simulink model "ThdRwRtStCalib"  (R2024b)
settings: Solver=FixedStepDiscrete  StartTime=0.0  StopTime=10.0  FixedStep=0.01  RelTol=1e-3
model workspace (MAT data in the model file):
  KeSMSwAcsMd7ThdRwRtStBkReclnUpwdDnwdPosMax_Val : Simulink.Parameter (value not decoded)
  KeSMSwAcsMd7ThdRwRtStBkReclnUpwdDnwdPosMin_Val : Simulink.Parameter (value not decoded)
  KeSMSwAcsMd7ThdRwRtStBkReclnUpwdDnwdPos_Val : Simulink.Parameter (value not decoded)
  KeSMSwAcsMd7ThdRwRtStCshnFldUpwdDnwdPosMax_Val : Simulink.Parameter (value not decoded)
  KeSMSwAcsMd7ThdRwRtStCshnFldUpwdDnwdPosMin_Val : Simulink.Parameter (value not decoded)
  KeSMSwAcsMd7ThdRwRtStCshnFldUpwdDnwdPos_Val : Simulink.Parameter (value not decoded)
  KeSMSwAcsMd7ThdRwRtStFrwdBkwdPosMax_Val : Simulink.Parameter (value not decoded)
  KeSMSwAcsMd7ThdRwRtStFrwdBkwdPosMin_Val : Simulink.Parameter (value not decoded)
  KeSMSwAcsMd7ThdRwRtStFrwdBkwdPos_Val : Simulink.Parameter (value not decoded)
symbols that are objects in the model workspace (value not decoded): KeSMSwAcsMd7ThdRwRtStBkReclnUpwdDnwdPos_Val, KeSMSwAcsMd7ThdRwRtStBkReclnUpwdDnwdPosMax_Val, KeSMSwAcsMd7ThdRwRtStBkReclnUpwdDnwdPosMin_Val, KeSMSwAcsMd7ThdRwRtStCshnFldUpwdDnwdPos_Val, KeSMSwAcsMd7ThdRwRtStCshnFldUpwdDnwdPosMax_Val, KeSMSwAcsMd7ThdRwRtStCshnFldUpwdDnwdPosMin_Val, KeSMSwAcsMd7ThdRwRtStFrwdBkwdPos_Val, KeSMSwAcsMd7ThdRwRtStFrwdBkwdPosMax_Val, KeSMSwAcsMd7ThdRwRtStFrwdBkwdPosMin_Val
undefined symbols (not defined in the file or in its folder): KeSMSw6sAcsEntryThdRwRtStBkReclnUpwdDnwdPos_Val, KeSMSw6sAcsEntryThdRwRtStBkReclnUpwdDnwdPosMax_Val, KeSMSw6sAcsEntryThdRwRtStBkReclnUpwdDnwdPosMin_Val, KeSMSw6sAcsEntryThdRwRtStCshnFldUpwdDnwdPos_Val, KeSMSw6sAcsEntryThdRwRtStCshnFldUpwdDnwdPosMax_Val, KeSMSw6sAcsEntryThdRwRtStCshnFldUpwdDnwdPosMin_Val, KeSMSw6sAcsEntryThdRwRtStFrwdBkwdPos_Val, KeSMSw6sAcsEntryThdRwRtStFrwdBkwdPosMax_Val, KeSMSw6sAcsEntryThdRwRtStFrwdBkwdPosMin_Val, KeSMSw6SAcsMd56ThdRwRtStBkReclnUpwdDnwdPos_Val, KeSMSw6SAcsMd56ThdRwRtStBkReclnUpwdDnwdPosMax_Val, KeSMSw6SAcsMd56ThdRwRtStBkReclnUpwdDnwdPosMin_Val, KeSMSw6SAcsMd56ThdRwRtStFrwdBkwdPos_Val, KeSMSw6SAcsMd56ThdRwRtStFrwdBkwdPosMax_Val, KeSMSw6SAcsMd56ThdRwRtStFrwdBkwdPosMin_Val, KeSMSw6SAcsMd57ThdRwRtStBkReclnUpwdDnwdPos_Val, KeSMSw6SAcsMd57ThdRwRtStBkReclnUpwdDnwdPosMax_Val, KeSMSw6SAcsMd57ThdRwRtStBkReclnUpwdDnwdPosMin_Val, KeSMSw6SAcsMd57ThdRwRtStFrwdBkwdPos_Val, KeSMSw6SAcsMd57ThdRwRtStFrwdBkwdPosMax_Val, KeSMSw6SAcsMd57ThdRwRtStFrwdBkwdPosMin_Val, KeSMSw6sFamilyMdThdRwRtStFrwdBkwdPos_Val, KeSMSw6sFamilyMdThdRwRtStFrwdBkwdPosMax_Val, KeSMSw6sFamilyMdThdRwRtStFrwdBkwdPosMin_Val, KeSMSw6sFamilyRMdThdRwRtStFrwdBkwdPos_Val, KeSMSw6sFamilyRMdThdRwRtStFrwdBkwdPosMax_Val, KeSMSw6sFamilyRMdThdRwRtStFrwdBkwdPosMin_Val, KeSMSw6sLugThdRwRtStBkReclnUpwdDnwdPos_Val, KeSMSw6sLugThdRwRtStBkReclnUpwdDnwdPosMax_Val, KeSMSw6sLugThdRwRtStBkReclnUpwdDnwdPosMin_Val, KeSMSw6sLugThdRwRtStCshnFldUpwdDnwdPos_Val, KeSMSw6sLugThdRwRtStCshnFldUpwdDnwdPosMax_Val, KeSMSw6sLugThdRwRtStCshnFldUpwdDnwdPosMin_Val, KeSMSw6sLugThdRwRtStFrwdBkwdPos_Val, KeSMSw6sLugThdRwRtStFrwdBkwdPosMax_Val, KeSMSw6sLugThdRwRtStFrwdBkwdPosMin_Val, KeSMSw6sVIPThdRwRtStBkReclnUpwdDnwdPos_Val, KeSMSw6sVIPThdRwRtStBkReclnUpwdDnwdPosMax_Val, KeSMSw6sVIPThdRwRtStBkReclnUpwdDnwdPosMin_Val, KeSMSw6sVIPThdRwRtStFrwdBkwdPos_Val, KeSMSw6sVIPThdRwRtStFrwdBkwdPosMax_Val, KeSMSw6sVIPThdRwRtStFrwdBkwdPosMin_Val, KeSMSwAcsEntryThdRwRtStBkReclnUpwdDnwdPos_Val, KeSMSwAcsEntryThdRwRtStBkReclnUpwdDnwdPosMax_Val, KeSMSwAcsEntryThdRwRtStBkReclnUpwdDnwdPosMin_Val, KeSMSwAcsEntryThdRwRtStCshnFldUpwdDnwdPos_Val, KeSMSwAcsEntryThdRwRtStCshnFldUpwdDnwdPosMax_Val, KeSMSwAcsEntryThdRwRtStCshnFldUpwdDnwdPosMin_Val, KeSMSwAcsEntryThdRwRtStFrwdBkwdPos_Val, KeSMSwAcsEntryThdRwRtStFrwdBkwdPosMax_Val, KeSMSwAcsEntryThdRwRtStFrwdBkwdPosMin_Val, KeSMSwAcsMd53ThdRwRtBkReclnUpwdDnwdPos_Val, KeSMSwAcsMd53ThdRwRtBkReclnUpwdDnwdPosMax_Val, KeSMSwAcsMd53ThdRwRtBkReclnUpwdDnwdPosMin_Val, KeSMSwAcsMd53ThdRwRtFldUpwdDnwdPos_Val, KeSMSwAcsMd53ThdRwRtFldUpwdDnwdPosMax_Val, KeSMSwAcsMd53ThdRwRtFldUpwdDnwdPosMin_Val, KeSMSwAcsMd56ThdRwRtStBkReclnUpwdDnwdPos_Val, KeSMSwAcsMd56ThdRwRtStBkReclnUpwdDnwdPosMax_Val, KeSMSwAcsMd56ThdRwRtStBkReclnUpwdDnwdPosMin_Val ... (+33)
libraries: TrgtPosSelcLib x18
(part 2 of 3)

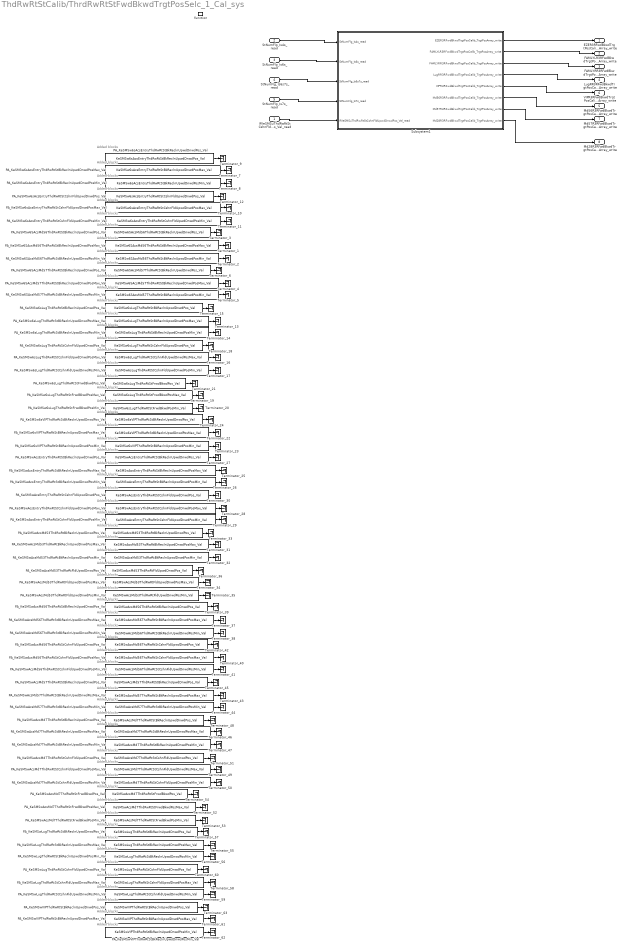
== system ThdRwRtStCalib/ThrdRwRtStFwdBkwdTrgtPosSelc_1_Cal_sys ==
  note: Added blocks
  note: Added blocks
  note: Added blocks
  note: Added blocks
  note: Added blocks
  note: Added blocks
  note: Added blocks
  note: Added blocks
  note: Added blocks
  note: Added blocks
  note: Added blocks
  note: Added blocks
  note: Added blocks
  note: Added blocks
  note: Added blocks
  note: Added blocks
  note: Added blocks
  note: Added blocks
  note: Added blocks
  note: Added blocks
  note: Added blocks
  note: Added blocks
  note: Added blocks
  note: Added blocks
  note: Added blocks
  note: Added blocks
  note: Added blocks
  note: Added blocks
  note: Added blocks
  note: Added blocks
  note: Added blocks
  note: Added blocks
  note: Added blocks
  note: Added blocks
  note: Added blocks
  note: Added blocks
  note: Added blocks
  note: Added blocks
  note: Added blocks
  note: Added blocks
  note: Added blocks
  note: Added blocks
  note: Added blocks
  note: Added blocks
  note: Added blocks
  note: Added blocks
  note: Added blocks
  note: Added blocks
  note: Added blocks
  note: Added blocks
  note: Added blocks
  note: Added blocks
  note: Added blocks
  note: Added blocks
  note: Added blocks
  note: Added blocks
  note: Added blocks
  note: Added blocks
  note: Added blocks
  note: Added blocks
  note: Added blocks
  note: Added blocks
  note: Added blocks
  IfVeSMSuThdRwRtStCshnFldUpwdDnwdPos_Val_read : Inport
  StNumFlg_Is4s_read : Inport  Port=2
  StNumFlg_Is6s_read : Inport  Port=3
  StNumFlg_Is6s7s_read : Inport  Port=4
  StNumFlg_Is7s_read : Inport  Port=5
  function : TriggerPort  TriggerType=function-call  IsSimulinkFunction=on  FunctionName=ThrdRwRtStFwdBkwdTrgtPosSelc_1_Cal  VariantControl=(inherit)
  PA_KeSMSw6SAcsMd56ThdRwRtStBkReclnUpwdDnwdPosMax_Val : Constant  Value=KeSMSw6SAcsMd56ThdRwRtStBkReclnUpwdDnwdPosMax_Val
  PA_KeSMSw6SAcsMd56ThdRwRtStBkReclnUpwdDnwdPosMin_Val : Constant  Value=KeSMSw6SAcsMd56ThdRwRtStBkReclnUpwdDnwdPosMin_Val
  PA_KeSMSw6SAcsMd56ThdRwRtStBkReclnUpwdDnwdPos_Val : Constant  Value=KeSMSw6SAcsMd56ThdRwRtStBkReclnUpwdDnwdPos_Val
  PA_KeSMSw6SAcsMd57ThdRwRtStBkReclnUpwdDnwdPosMax_Val : Constant  Value=KeSMSw6SAcsMd57ThdRwRtStBkReclnUpwdDnwdPosMax_Val
  PA_KeSMSw6SAcsMd57ThdRwRtStBkReclnUpwdDnwdPosMin_Val : Constant  Value=KeSMSw6SAcsMd57ThdRwRtStBkReclnUpwdDnwdPosMin_Val
  PA_KeSMSw6SAcsMd57ThdRwRtStBkReclnUpwdDnwdPos_Val : Constant  Value=KeSMSw6SAcsMd57ThdRwRtStBkReclnUpwdDnwdPos_Val
  PA_KeSMSw6sAcsEntryThdRwRtStBkReclnUpwdDnwdPosMax_Val : Constant  Value=KeSMSw6sAcsEntryThdRwRtStBkReclnUpwdDnwdPosMax_Val
  PA_KeSMSw6sAcsEntryThdRwRtStBkReclnUpwdDnwdPosMin_Val : Constant  Value=KeSMSw6sAcsEntryThdRwRtStBkReclnUpwdDnwdPosMin_Val
  PA_KeSMSw6sAcsEntryThdRwRtStBkReclnUpwdDnwdPos_Val : Constant  Value=KeSMSw6sAcsEntryThdRwRtStBkReclnUpwdDnwdPos_Val
  PA_KeSMSw6sAcsEntryThdRwRtStCshnFldUpwdDnwdPosMax_Val : Constant  Value=KeSMSw6sAcsEntryThdRwRtStCshnFldUpwdDnwdPosMax_Val
  PA_KeSMSw6sAcsEntryThdRwRtStCshnFldUpwdDnwdPosMin_Val : Constant  Value=KeSMSw6sAcsEntryThdRwRtStCshnFldUpwdDnwdPosMin_Val
  PA_KeSMSw6sAcsEntryThdRwRtStCshnFldUpwdDnwdPos_Val : Constant  Value=KeSMSw6sAcsEntryThdRwRtStCshnFldUpwdDnwdPos_Val
  PA_KeSMSw6sLugThdRwRtStBkReclnUpwdDnwdPosMax_Val : Constant  Value=KeSMSw6sLugThdRwRtStBkReclnUpwdDnwdPosMax_Val
  PA_KeSMSw6sLugThdRwRtStBkReclnUpwdDnwdPosMin_Val : Constant  Value=KeSMSw6sLugThdRwRtStBkReclnUpwdDnwdPosMin_Val
  PA_KeSMSw6sLugThdRwRtStBkReclnUpwdDnwdPos_Val : Constant  Value=KeSMSw6sLugThdRwRtStBkReclnUpwdDnwdPos_Val
  PA_KeSMSw6sLugThdRwRtStCshnFldUpwdDnwdPosMax_Val : Constant  Value=KeSMSw6sLugThdRwRtStCshnFldUpwdDnwdPosMax_Val
  PA_KeSMSw6sLugThdRwRtStCshnFldUpwdDnwdPosMin_Val : Constant  Value=KeSMSw6sLugThdRwRtStCshnFldUpwdDnwdPosMin_Val
  PA_KeSMSw6sLugThdRwRtStCshnFldUpwdDnwdPos_Val : Constant  Value=KeSMSw6sLugThdRwRtStCshnFldUpwdDnwdPos_Val
  PA_KeSMSw6sLugThdRwRtStFrwdBkwdPosMax_Val : Constant  Value=KeSMSw6sLugThdRwRtStFrwdBkwdPosMax_Val
  PA_KeSMSw6sLugThdRwRtStFrwdBkwdPosMin_Val : Constant  Value=KeSMSw6sLugThdRwRtStFrwdBkwdPosMin_Val
  PA_KeSMSw6sLugThdRwRtStFrwdBkwdPos_Val : Constant  Value=KeSMSw6sLugThdRwRtStFrwdBkwdPos_Val
  PA_KeSMSw6sVIPThdRwRtStBkReclnUpwdDnwdPosMax_Val : Constant  Value=KeSMSw6sVIPThdRwRtStBkReclnUpwdDnwdPosMax_Val
  PA_KeSMSw6sVIPThdRwRtStBkReclnUpwdDnwdPosMin_Val : Constant  Value=KeSMSw6sVIPThdRwRtStBkReclnUpwdDnwdPosMin_Val
  PA_KeSMSw6sVIPThdRwRtStBkReclnUpwdDnwdPos_Val : Constant  Value=KeSMSw6sVIPThdRwRtStBkReclnUpwdDnwdPos_Val
  PA_KeSMSwAcsEntryThdRwRtStBkReclnUpwdDnwdPosMax_Val : Constant  Value=KeSMSwAcsEntryThdRwRtStBkReclnUpwdDnwdPosMax_Val
  PA_KeSMSwAcsEntryThdRwRtStBkReclnUpwdDnwdPosMin_Val : Constant  Value=KeSMSwAcsEntryThdRwRtStBkReclnUpwdDnwdPosMin_Val
  PA_KeSMSwAcsEntryThdRwRtStBkReclnUpwdDnwdPos_Val : Constant  Value=KeSMSwAcsEntryThdRwRtStBkReclnUpwdDnwdPos_Val
  PA_KeSMSwAcsEntryThdRwRtStCshnFldUpwdDnwdPosMax_Val : Constant  Value=KeSMSwAcsEntryThdRwRtStCshnFldUpwdDnwdPosMax_Val
  PA_KeSMSwAcsEntryThdRwRtStCshnFldUpwdDnwdPosMin_Val : Constant  Value=KeSMSwAcsEntryThdRwRtStCshnFldUpwdDnwdPosMin_Val
  PA_KeSMSwAcsEntryThdRwRtStCshnFldUpwdDnwdPos_Val : Constant  Value=KeSMSwAcsEntryThdRwRtStCshnFldUpwdDnwdPos_Val
  PA_KeSMSwAcsMd53ThdRwRtBkReclnUpwdDnwdPosMax_Val : Constant  Value=KeSMSwAcsMd53ThdRwRtBkReclnUpwdDnwdPosMax_Val
  PA_KeSMSwAcsMd53ThdRwRtBkReclnUpwdDnwdPosMin_Val : Constant  Value=KeSMSwAcsMd53ThdRwRtBkReclnUpwdDnwdPosMin_Val
  PA_KeSMSwAcsMd53ThdRwRtBkReclnUpwdDnwdPos_Val : Constant  Value=KeSMSwAcsMd53ThdRwRtBkReclnUpwdDnwdPos_Val
  PA_KeSMSwAcsMd53ThdRwRtFldUpwdDnwdPosMax_Val : Constant  Value=KeSMSwAcsMd53ThdRwRtFldUpwdDnwdPosMax_Val
  PA_KeSMSwAcsMd53ThdRwRtFldUpwdDnwdPosMin_Val : Constant  Value=KeSMSwAcsMd53ThdRwRtFldUpwdDnwdPosMin_Val
  PA_KeSMSwAcsMd53ThdRwRtFldUpwdDnwdPos_Val : Constant  Value=KeSMSwAcsMd53ThdRwRtFldUpwdDnwdPos_Val
  PA_KeSMSwAcsMd56ThdRwRtStBkReclnUpwdDnwdPosMax_Val : Constant  Value=KeSMSwAcsMd56ThdRwRtStBkReclnUpwdDnwdPosMax_Val
  PA_KeSMSwAcsMd56ThdRwRtStBkReclnUpwdDnwdPosMin_Val : Constant  Value=KeSMSwAcsMd56ThdRwRtStBkReclnUpwdDnwdPosMin_Val
  PA_KeSMSwAcsMd56ThdRwRtStBkReclnUpwdDnwdPos_Val : Constant  Value=KeSMSwAcsMd56ThdRwRtStBkReclnUpwdDnwdPos_Val
  PA_KeSMSwAcsMd56ThdRwRtStCshnFldUpwdDnwdPosMax_Val : Constant  Value=KeSMSwAcsMd56ThdRwRtStCshnFldUpwdDnwdPosMax_Val
  PA_KeSMSwAcsMd56ThdRwRtStCshnFldUpwdDnwdPosMin_Val : Constant  Value=KeSMSwAcsMd56ThdRwRtStCshnFldUpwdDnwdPosMin_Val
  PA_KeSMSwAcsMd56ThdRwRtStCshnFldUpwdDnwdPos_Val : Constant  Value=KeSMSwAcsMd56ThdRwRtStCshnFldUpwdDnwdPos_Val
  PA_KeSMSwAcsMd57ThdRwRtStBkReclnUpwdDnwdPosMax_Val : Constant  Value=KeSMSwAcsMd57ThdRwRtStBkReclnUpwdDnwdPosMax_Val
  PA_KeSMSwAcsMd57ThdRwRtStBkReclnUpwdDnwdPosMin_Val : Constant  Value=KeSMSwAcsMd57ThdRwRtStBkReclnUpwdDnwdPosMin_Val
  PA_KeSMSwAcsMd57ThdRwRtStBkReclnUpwdDnwdPos_Val : Constant  Value=KeSMSwAcsMd57ThdRwRtStBkReclnUpwdDnwdPos_Val
  PA_KeSMSwAcsMd7ThdRwRtStBkReclnUpwdDnwdPosMax_Val : Constant  Value=KeSMSwAcsMd7ThdRwRtStBkReclnUpwdDnwdPosMax_Val
  PA_KeSMSwAcsMd7ThdRwRtStBkReclnUpwdDnwdPosMin_Val : Constant  Value=KeSMSwAcsMd7ThdRwRtStBkReclnUpwdDnwdPosMin_Val
  PA_KeSMSwAcsMd7ThdRwRtStBkReclnUpwdDnwdPos_Val : Constant  Value=KeSMSwAcsMd7ThdRwRtStBkReclnUpwdDnwdPos_Val
  PA_KeSMSwAcsMd7ThdRwRtStCshnFldUpwdDnwdPosMax_Val : Constant  Value=KeSMSwAcsMd7ThdRwRtStCshnFldUpwdDnwdPosMax_Val
  PA_KeSMSwAcsMd7ThdRwRtStCshnFldUpwdDnwdPosMin_Val : Constant  Value=KeSMSwAcsMd7ThdRwRtStCshnFldUpwdDnwdPosMin_Val
  PA_KeSMSwAcsMd7ThdRwRtStCshnFldUpwdDnwdPos_Val : Constant  Value=KeSMSwAcsMd7ThdRwRtStCshnFldUpwdDnwdPos_Val
  PA_KeSMSwAcsMd7ThdRwRtStFrwdBkwdPosMax_Val : Constant  Value=KeSMSwAcsMd7ThdRwRtStFrwdBkwdPosMax_Val
  PA_KeSMSwAcsMd7ThdRwRtStFrwdBkwdPosMin_Val : Constant  Value=KeSMSwAcsMd7ThdRwRtStFrwdBkwdPosMin_Val
  PA_KeSMSwAcsMd7ThdRwRtStFrwdBkwdPos_Val : Constant  Value=KeSMSwAcsMd7ThdRwRtStFrwdBkwdPos_Val
  PA_KeSMSwLugThdRwRtStBkReclnUpwdDnwdPosMax_Val : Constant  Value=KeSMSwLugThdRwRtStBkReclnUpwdDnwdPosMax_Val
  PA_KeSMSwLugThdRwRtStBkReclnUpwdDnwdPosMin_Val : Constant  Value=KeSMSwLugThdRwRtStBkReclnUpwdDnwdPosMin_Val
  PA_KeSMSwLugThdRwRtStBkReclnUpwdDnwdPos_Val : Constant  Value=KeSMSwLugThdRwRtStBkReclnUpwdDnwdPos_Val
  PA_KeSMSwLugThdRwRtStCshnFldUpwdDnwdPosMax_Val : Constant  Value=KeSMSwLugThdRwRtStCshnFldUpwdDnwdPosMax_Val
  PA_KeSMSwLugThdRwRtStCshnFldUpwdDnwdPosMin_Val : Constant  Value=KeSMSwLugThdRwRtStCshnFldUpwdDnwdPosMin_Val
  PA_KeSMSwLugThdRwRtStCshnFldUpwdDnwdPos_Val : Constant  Value=KeSMSwLugThdRwRtStCshnFldUpwdDnwdPos_Val
  PA_KeSMSwVIPThdRwRtStBkReclnUpwdDnwdPosMax_Val : Constant  Value=KeSMSwVIPThdRwRtStBkReclnUpwdDnwdPosMax_Val
  PA_KeSMSwVIPThdRwRtStBkReclnUpwdDnwdPosMin_Val : Constant  Value=KeSMSwVIPThdRwRtStBkReclnUpwdDnwdPosMin_Val
  PA_KeSMSwVIPThdRwRtStBkReclnUpwdDnwdPos_Val : Constant  Value=KeSMSwVIPThdRwRtStBkReclnUpwdDnwdPos_Val
  Subsystem1 : Subsystem
  Terminator_{1..63} (63 alike) : Terminator
  EZER3RFwdBkwdTrgtPosCalib_TrgtPosArray_write : Outport  VectorParamsAs1DForOutWhenUnconnected=off
  FAMLYLR3RFwdBkwdTrgtPosCalib_TrgtPosArray_write : Outport  Port=2  VectorParamsAs1DForOutWhenUnconnected=off
  FAMLYRR3RFwdBkwdTrgtPosCalib_TrgtPosArray_write : Outport  Port=3  VectorParamsAs1DForOutWhenUnconnected=off
  LugRR3RFwdBkwdTrgtPosCalib_TrgtPosArray_write : Outport  Port=4  VectorParamsAs1DForOutWhenUnconnected=off
  Md56R3RFwdBkwdTrgtPosCalib_TrgtPosArray_write : Outport  Port=5  VectorParamsAs1DForOutWhenUnconnected=off
  VIPR3RFwdBkwdTrgtPosCalib_TrgtPosArray_write : Outport  Port=6  VectorParamsAs1DForOutWhenUnconnected=off
  Md57R3RFwdBkwdTrgtPosCalib_TrgtPosArray_write : Outport  Port=7  VectorParamsAs1DForOutWhenUnconnected=off
  Md28R3RFwdBkwdTrgtPosCalib_TrgtPosArray_write : Outport  Port=8  VectorParamsAs1DForOutWhenUnconnected=off
      settings: EnsureOutportIsVirtual=on
  wires:
  Subsystem1/1(EZER3RFwdBkwdTrgtPosCalib_TrgtPosArray_write) -> EZER3RFwdBkwdTrgtPosCalib_TrgtPosArray_write/1
  Subsystem1/2(FAMLYLR3RFwdBkwdTrgtPosCalib_TrgtPosArray_write) -> FAMLYLR3RFwdBkwdTrgtPosCalib_TrgtPosArray_write/1
  Subsystem1/3(FAMLYRR3RFwdBkwdTrgtPosCalib_TrgtPosArray_write) -> FAMLYRR3RFwdBkwdTrgtPosCalib_TrgtPosArray_write/1
  Subsystem1/4(LugRR3RFwdBkwdTrgtPosCalib_TrgtPosArray_write) -> LugRR3RFwdBkwdTrgtPosCalib_TrgtPosArray_write/1
  Subsystem1/5(VIPR3RFwdBkwdTrgtPosCalib_TrgtPosArray_write) -> VIPR3RFwdBkwdTrgtPosCalib_TrgtPosArray_write/1
  Subsystem1/6(Md56R3RFwdBkwdTrgtPosCalib_TrgtPosArray_write) -> Md56R3RFwdBkwdTrgtPosCalib_TrgtPosArray_write/1
  Subsystem1/7(Md57R3RFwdBkwdTrgtPosCalib_TrgtPosArray_write) -> Md57R3RFwdBkwdTrgtPosCalib_TrgtPosArray_write/1
  StNumFlg_Is4s_read/1 -> Subsystem1/1(StNumFlg_Is4s_read)
  StNumFlg_Is6s_read/1 -> Subsystem1/2(StNumFlg_Is6s_read)
  StNumFlg_Is6s7s_read/1 -> Subsystem1/3(StNumFlg_Is6s7s_read)
  StNumFlg_Is7s_read/1 -> Subsystem1/4(StNumFlg_Is7s_read)
  IfVeSMSuThdRwRtStCshnFldUpwdDnwdPos_Val_read/1 -> Subsystem1/5(IfVeSMSuThdRwRtStCshnFldUpwdDnwdPos_Val_read)
  Subsystem1/8(Md28R3RFwdBkwdTrgtPosCalib_TrgtPosArray_write) -> Md28R3RFwdBkwdTrgtPosCalib_TrgtPosArray_write/1
  PA_KeSMSw6SAcsMd56ThdRwRtStBkReclnUpwdDnwdPosMax_Val/1 -> Terminator_1/1
  PA_KeSMSw6SAcsMd56ThdRwRtStBkReclnUpwdDnwdPosMin_Val/1 -> Terminator_2/1
  PA_KeSMSw6SAcsMd56ThdRwRtStBkReclnUpwdDnwdPos_Val/1 -> Terminator_3/1
  PA_KeSMSw6SAcsMd57ThdRwRtStBkReclnUpwdDnwdPosMax_Val/1 -> Terminator_4/1
  PA_KeSMSw6SAcsMd57ThdRwRtStBkReclnUpwdDnwdPosMin_Val/1 -> Terminator_5/1
  PA_KeSMSw6SAcsMd57ThdRwRtStBkReclnUpwdDnwdPos_Val/1 -> Terminator_6/1
  PA_KeSMSw6sAcsEntryThdRwRtStBkReclnUpwdDnwdPosMax_Val/1 -> Terminator_7/1
  PA_KeSMSw6sAcsEntryThdRwRtStBkReclnUpwdDnwdPosMin_Val/1 -> Terminator_8/1
  PA_KeSMSw6sAcsEntryThdRwRtStBkReclnUpwdDnwdPos_Val/1 -> Terminator_9/1
  PA_KeSMSw6sAcsEntryThdRwRtStCshnFldUpwdDnwdPosMax_Val/1 -> Terminator_10/1
  PA_KeSMSw6sAcsEntryThdRwRtStCshnFldUpwdDnwdPosMin_Val/1 -> Terminator_11/1
  PA_KeSMSw6sAcsEntryThdRwRtStCshnFldUpwdDnwdPos_Val/1 -> Terminator_12/1
  PA_KeSMSw6sLugThdRwRtStBkReclnUpwdDnwdPosMax_Val/1 -> Terminator_13/1
  PA_KeSMSw6sLugThdRwRtStBkReclnUpwdDnwdPosMin_Val/1 -> Terminator_14/1
  PA_KeSMSw6sLugThdRwRtStBkReclnUpwdDnwdPos_Val/1 -> Terminator_15/1
  PA_KeSMSw6sLugThdRwRtStCshnFldUpwdDnwdPosMax_Val/1 -> Terminator_16/1
  PA_KeSMSw6sLugThdRwRtStCshnFldUpwdDnwdPosMin_Val/1 -> Terminator_17/1
  PA_KeSMSw6sLugThdRwRtStCshnFldUpwdDnwdPos_Val/1 -> Terminator_18/1
  PA_KeSMSw6sLugThdRwRtStFrwdBkwdPosMax_Val/1 -> Terminator_19/1
  PA_KeSMSw6sLugThdRwRtStFrwdBkwdPosMin_Val/1 -> Terminator_20/1
  PA_KeSMSw6sLugThdRwRtStFrwdBkwdPos_Val/1 -> Terminator_21/1
  PA_KeSMSw6sVIPThdRwRtStBkReclnUpwdDnwdPosMax_Val/1 -> Terminator_22/1
  PA_KeSMSw6sVIPThdRwRtStBkReclnUpwdDnwdPosMin_Val/1 -> Terminator_23/1
  PA_KeSMSw6sVIPThdRwRtStBkReclnUpwdDnwdPos_Val/1 -> Terminator_24/1
  PA_KeSMSwAcsEntryThdRwRtStBkReclnUpwdDnwdPosMax_Val/1 -> Terminator_25/1
  PA_KeSMSwAcsEntryThdRwRtStBkReclnUpwdDnwdPosMin_Val/1 -> Terminator_26/1
  PA_KeSMSwAcsEntryThdRwRtStBkReclnUpwdDnwdPos_Val/1 -> Terminator_27/1
  PA_KeSMSwAcsEntryThdRwRtStCshnFldUpwdDnwdPosMax_Val/1 -> Terminator_28/1
  PA_KeSMSwAcsEntryThdRwRtStCshnFldUpwdDnwdPosMin_Val/1 -> Terminator_29/1
  PA_KeSMSwAcsEntryThdRwRtStCshnFldUpwdDnwdPos_Val/1 -> Terminator_30/1
  PA_KeSMSwAcsMd53ThdRwRtBkReclnUpwdDnwdPosMax_Val/1 -> Terminator_31/1
  PA_KeSMSwAcsMd53ThdRwRtBkReclnUpwdDnwdPosMin_Val/1 -> Terminator_32/1
  PA_KeSMSwAcsMd53ThdRwRtBkReclnUpwdDnwdPos_Val/1 -> Terminator_33/1
  PA_KeSMSwAcsMd53ThdRwRtFldUpwdDnwdPosMax_Val/1 -> Terminator_34/1
  PA_KeSMSwAcsMd53ThdRwRtFldUpwdDnwdPosMin_Val/1 -> Terminator_35/1
  PA_KeSMSwAcsMd53ThdRwRtFldUpwdDnwdPos_Val/1 -> Terminator_36/1
  PA_KeSMSwAcsMd56ThdRwRtStBkReclnUpwdDnwdPosMax_Val/1 -> Terminator_37/1
  PA_KeSMSwAcsMd56ThdRwRtStBkReclnUpwdDnwdPosMin_Val/1 -> Terminator_38/1
  PA_KeSMSwAcsMd56ThdRwRtStBkReclnUpwdDnwdPos_Val/1 -> Terminator_39/1
  PA_KeSMSwAcsMd56ThdRwRtStCshnFldUpwdDnwdPosMax_Val/1 -> Terminator_40/1
  PA_KeSMSwAcsMd56ThdRwRtStCshnFldUpwdDnwdPosMin_Val/1 -> Terminator_41/1
  PA_KeSMSwAcsMd56ThdRwRtStCshnFldUpwdDnwdPos_Val/1 -> Terminator_42/1
  PA_KeSMSwAcsMd57ThdRwRtStBkReclnUpwdDnwdPosMax_Val/1 -> Terminator_43/1
  PA_KeSMSwAcsMd57ThdRwRtStBkReclnUpwdDnwdPosMin_Val/1 -> Terminator_44/1
  PA_KeSMSwAcsMd57ThdRwRtStBkReclnUpwdDnwdPos_Val/1 -> Terminator_45/1
  PA_KeSMSwAcsMd7ThdRwRtStBkReclnUpwdDnwdPosMax_Val/1 -> Terminator_46/1
  PA_KeSMSwAcsMd7ThdRwRtStBkReclnUpwdDnwdPosMin_Val/1 -> Terminator_47/1
  PA_KeSMSwAcsMd7ThdRwRtStBkReclnUpwdDnwdPos_Val/1 -> Terminator_48/1
  PA_KeSMSwAcsMd7ThdRwRtStCshnFldUpwdDnwdPosMax_Val/1 -> Terminator_49/1
  PA_KeSMSwAcsMd7ThdRwRtStCshnFldUpwdDnwdPosMin_Val/1 -> Terminator_50/1
  PA_KeSMSwAcsMd7ThdRwRtStCshnFldUpwdDnwdPos_Val/1 -> Terminator_51/1
  PA_KeSMSwAcsMd7ThdRwRtStFrwdBkwdPosMax_Val/1 -> Terminator_52/1
  PA_KeSMSwAcsMd7ThdRwRtStFrwdBkwdPosMin_Val/1 -> Terminator_53/1
  PA_KeSMSwAcsMd7ThdRwRtStFrwdBkwdPos_Val/1 -> Terminator_54/1
  PA_KeSMSwLugThdRwRtStBkReclnUpwdDnwdPosMax_Val/1 -> Terminator_55/1
  PA_KeSMSwLugThdRwRtStBkReclnUpwdDnwdPosMin_Val/1 -> Terminator_56/1
  PA_KeSMSwLugThdRwRtStBkReclnUpwdDnwdPos_Val/1 -> Terminator_57/1
  PA_KeSMSwLugThdRwRtStCshnFldUpwdDnwdPosMax_Val/1 -> Terminator_58/1
  PA_KeSMSwLugThdRwRtStCshnFldUpwdDnwdPosMin_Val/1 -> Terminator_59/1
  PA_KeSMSwLugThdRwRtStCshnFldUpwdDnwdPos_Val/1 -> Terminator_60/1
  PA_KeSMSwVIPThdRwRtStBkReclnUpwdDnwdPosMax_Val/1 -> Terminator_61/1
  PA_KeSMSwVIPThdRwRtStBkReclnUpwdDnwdPosMin_Val/1 -> Terminator_62/1
  PA_KeSMSwVIPThdRwRtStBkReclnUpwdDnwdPos_Val/1 -> Terminator_63/1

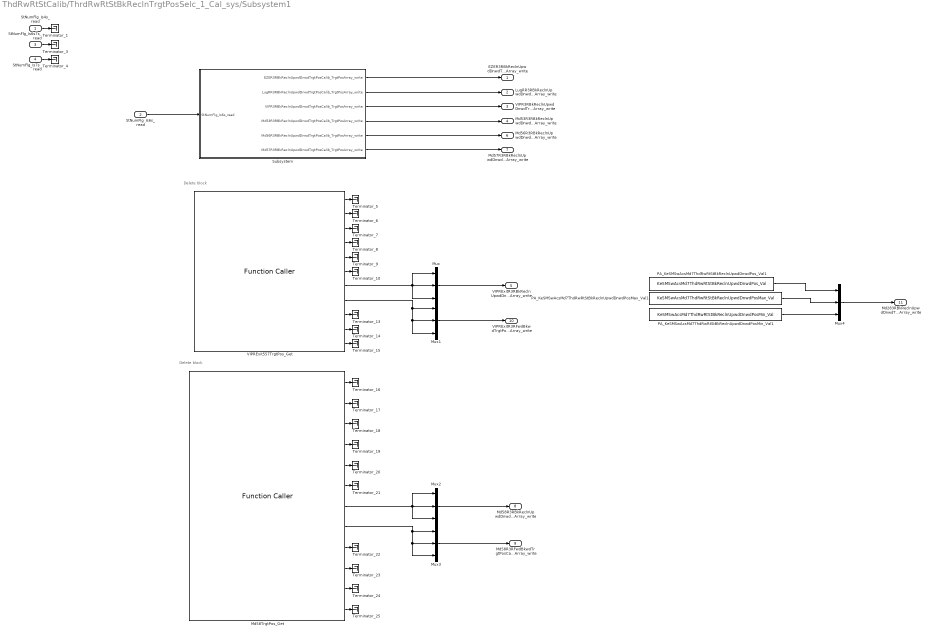
== system ThdRwRtStCalib/ThrdRwRtStBkReclnTrgtPosSelc_1_Cal_sys/Subsystem1 ==
  note: Delete block
  note: Delete block
  StNumFlg_Is4s_read : Inport
  StNumFlg_Is6s_read : Inport  Port=2
  StNumFlg_Is6s7s_read : Inport  Port=3
  StNumFlg_Is7s_read : Inport  Port=4
  Md58TrgtPos_Get : FunctionCaller  FunctionPrototype=[SecRwRtStBkReclnTrgtPos,SecRwRtStZeroTrgtPos,SecRwRtStLgrstUpwdDnwdTrgtPos,SecRwRtStLgrstInwdOtwdTrgtPos,ThdRwLtStBkReclnTrgtPos,ThdRwLtStFwdBkwdTrgtPos,ThdRwRtStBkReclnTrgtPos,ThdRwRtStFwdBkwdTrgtPos,PassStBkReclnTrgtPos,PassStFwdBkwdTrgtPos,SecRwRtStFwdBkwdTrgtPos,PassStFldTrgtPos] = Md58TrgtPos_Get()  InputArgumentSpecifications=<Enter example>  OutputArgumentSpecifications=uint16(1), uint16(1), uint16(1), uint16(1), uint16(1), uint16(1), uint16(1), uint16(1), uint16(1), uint16(1), uint16(1), uint16(1)
  Mux{,1..4} (5 alike) : Mux  Inputs=3
  PA_KeSMSwAcsMd7ThdRwRtStBkReclnUpwdDnwdPosMax_Val1 : Constant  Value=KeSMSwAcsMd7ThdRwRtStBkReclnUpwdDnwdPosMax_Val
  PA_KeSMSwAcsMd7ThdRwRtStBkReclnUpwdDnwdPosMin_Val1 : Constant  Value=KeSMSwAcsMd7ThdRwRtStBkReclnUpwdDnwdPosMin_Val
  PA_KeSMSwAcsMd7ThdRwRtStBkReclnUpwdDnwdPos_Val1 : Constant  Value=KeSMSwAcsMd7ThdRwRtStBkReclnUpwdDnwdPos_Val
  Subsystem : Subsystem
  Terminator_{1,3..10,13..25} (22 alike) : Terminator
  VIPRExit557TrgtPos_Get : FunctionCaller  FunctionPrototype=[SecRwRtStBkReclnTrgtPos,SecRwRtStZeroTrgtPos,SecRwRtStLgrstUpwdDnwdTrgtPos,SecRwRtStLgrstInwdOtwdTrgtPos,ThdRwLtStBkReclnTrgtPos,ThdRwLtStFwdBkwdTrgtPos,ThdRwRtStBkReclnTrgtPos,ThdRwRtStFwdBkwdTrgtPos,PassStBkReclnTrgtPos,PassStFwdBkwdTrgtPos,SecRwRtStFwdBkwdTrgtPos] = VIPRExit557TrgtPos_Get()  InputArgumentSpecifications=<Enter example>  OutputArgumentSpecifications=uint16(1), uint16(1), uint16(1), uint16(1), uint16(1), uint16(1), uint16(1), uint16(1), uint16(1), uint16(1), uint16(1)
  EZER3RBkReclnUpwdDnwdTrgtPosCalib_TrgtPosArray_write : Outport  VectorParamsAs1DForOutWhenUnconnected=off
      settings: EnsureOutportIsVirtual=on
  LugRR3RBkReclnUpwdDnwdTrgtPosCalib_TrgtPosArray_write : Outport  Port=2  VectorParamsAs1DForOutWhenUnconnected=off
      settings: EnsureOutportIsVirtual=on
  VIPR3RBkReclnUpwdDnwdTrgtPosCalib_TrgtPosArray_write : Outport  Port=3  VectorParamsAs1DForOutWhenUnconnected=off
      settings: EnsureOutportIsVirtual=on
  Md53R3RBkReclnUpwdDnwdTrgtPosCalib_TrgtPosArray_write : Outport  Port=4  VectorParamsAs1DForOutWhenUnconnected=off
      settings: EnsureOutportIsVirtual=on
  VIPRExitR3RBkReclnUpwdDnwdTrgtPosCalib_TrgtPosArray_write : Outport  Port=5  VectorParamsAs1DForOutWhenUnconnected=off
      settings: EnsureOutportIsVirtual=on
  Md56R3RBkReclnUpwdDnwdTrgtPosCalib_TrgtPosArray_write : Outport  Port=6  VectorParamsAs1DForOutWhenUnconnected=off
      settings: EnsureOutportIsVirtual=on
  Md57R3RBkReclnUpwdDnwdTrgtPosCalib_TrgtPosArray_write : Outport  Port=7  VectorParamsAs1DForOutWhenUnconnected=off
      settings: EnsureOutportIsVirtual=on
  Md58R3RBkReclnUpwdDnwdTrgtPosCalib_TrgtPosArray_write : Outport  Port=8  VectorParamsAs1DForOutWhenUnconnected=off
      settings: EnsureOutportIsVirtual=on
  Md58R3RFwdBkwdTrgtPosCalib_TrgtPosArray_write : Outport  Port=9  VectorParamsAs1DForOutWhenUnconnected=off
      settings: EnsureOutportIsVirtual=on
  VIPRExitR3RFwdBkwdTrgtPosCalib_TrgtPosArray_write : Outport  Port=10  VectorParamsAs1DForOutWhenUnconnected=off
      settings: EnsureOutportIsVirtual=on
  Md283RBkReclnUpwdDnwdTrgtPosCalib_TrgtPosArray_write : Outport  Port=11  VectorParamsAs1DForOutWhenUnconnected=off
  wires:
  Subsystem/1(EZER3RBkReclnUpwdDnwdTrgtPosCalib_TrgtPosArray_write) -> EZER3RBkReclnUpwdDnwdTrgtPosCalib_TrgtPosArray_write/1
  StNumFlg_Is4s_read/1 -> Terminator_1/1
  Subsystem/3(VIPR3RBkReclnUpwdDnwdTrgtPosCalib_TrgtPosArray_write) -> VIPR3RBkReclnUpwdDnwdTrgtPosCalib_TrgtPosArray_write/1
  StNumFlg_Is7s_read/1 -> Terminator_4/1
  Subsystem/2(LugRR3RBkReclnUpwdDnwdTrgtPosCalib_TrgtPosArray_write) -> LugRR3RBkReclnUpwdDnwdTrgtPosCalib_TrgtPosArray_write/1
  StNumFlg_Is6s_read/1 -> Subsystem/1(StNumFlg_Is6s_read)
  StNumFlg_Is6s7s_read/1 -> Terminator_3/1
  Subsystem/4(Md53R3RBkReclnUpwdDnwdTrgtPosCalib_TrgtPosArray_write) -> Md53R3RBkReclnUpwdDnwdTrgtPosCalib_TrgtPosArray_write/1
  VIPRExit557TrgtPos_Get/1 -> Terminator_5/1
  VIPRExit557TrgtPos_Get/2 -> Terminator_6/1
  VIPRExit557TrgtPos_Get/3 -> Terminator_7/1
  VIPRExit557TrgtPos_Get/4 -> Terminator_8/1
  VIPRExit557TrgtPos_Get/5 -> Terminator_9/1
  VIPRExit557TrgtPos_Get/6 -> Terminator_10/1
  VIPRExit557TrgtPos_Get/7 -> Mux/3, Mux/1, Mux/2
  VIPRExit557TrgtPos_Get/9 -> Terminator_13/1
  VIPRExit557TrgtPos_Get/10 -> Terminator_14/1
  Mux/1 -> VIPRExitR3RBkReclnUpwdDnwdTrgtPosCalib_TrgtPosArray_write/1
  VIPRExit557TrgtPos_Get/11 -> Terminator_15/1
  Subsystem/5(Md56R3RBkReclnUpwdDnwdTrgtPosCalib_TrgtPosArray_write) -> Md56R3RBkReclnUpwdDnwdTrgtPosCalib_TrgtPosArray_write/1
  Mux1/1 -> VIPRExitR3RFwdBkwdTrgtPosCalib_TrgtPosArray_write/1
  VIPRExit557TrgtPos_Get/8 -> Mux1/2, Mux1/3, Mux1/1
  Mux2/1 -> Md58R3RBkReclnUpwdDnwdTrgtPosCalib_TrgtPosArray_write/1
  Mux3/1 -> Md58R3RFwdBkwdTrgtPosCalib_TrgtPosArray_write/1
  Subsystem/6(Md57R3RBkReclnUpwdDnwdTrgtPosCalib_TrgtPosArray_write) -> Md57R3RBkReclnUpwdDnwdTrgtPosCalib_TrgtPosArray_write/1
  Md58TrgtPos_Get/7 -> Mux2/2, Mux2/1, Mux2/3
  Md58TrgtPos_Get/8 -> Mux3/3, Mux3/2, Mux3/1
  Md58TrgtPos_Get/1 -> Terminator_16/1
  Md58TrgtPos_Get/2 -> Terminator_17/1
  Md58TrgtPos_Get/3 -> Terminator_18/1
  Md58TrgtPos_Get/4 -> Terminator_19/1
  Md58TrgtPos_Get/5 -> Terminator_20/1
  Md58TrgtPos_Get/6 -> Terminator_21/1
  Md58TrgtPos_Get/9 -> Terminator_22/1
  Md58TrgtPos_Get/10 -> Terminator_23/1
  Md58TrgtPos_Get/11 -> Terminator_24/1
  Md58TrgtPos_Get/12 -> Terminator_25/1
  Mux4/1 -> Md283RBkReclnUpwdDnwdTrgtPosCalib_TrgtPosArray_write/1
  PA_KeSMSwAcsMd7ThdRwRtStBkReclnUpwdDnwdPosMin_Val1/1 -> Mux4/3
  PA_KeSMSwAcsMd7ThdRwRtStBkReclnUpwdDnwdPosMax_Val1/1 -> Mux4/2
  PA_KeSMSwAcsMd7ThdRwRtStBkReclnUpwdDnwdPos_Val1/1 -> Mux4/1

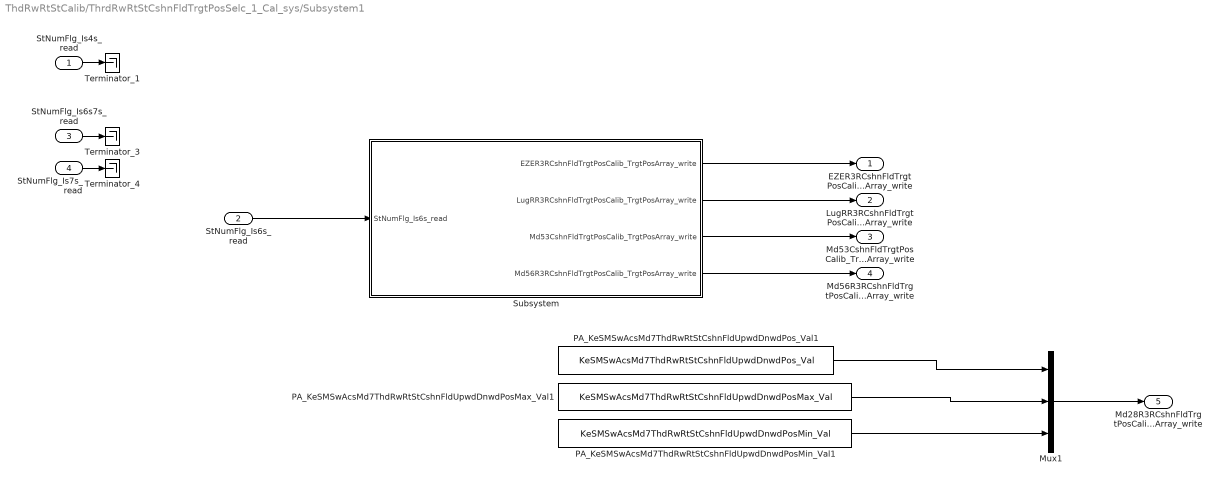
== system ThdRwRtStCalib/ThrdRwRtStCshnFldTrgtPosSelc_1_Cal_sys/Subsystem1 ==
  StNumFlg_Is4s_read : Inport
  StNumFlg_Is6s_read : Inport  Port=2
  StNumFlg_Is6s7s_read : Inport  Port=3
  StNumFlg_Is7s_read : Inport  Port=4
  Mux1 : Mux  Inputs=3
  PA_KeSMSwAcsMd7ThdRwRtStCshnFldUpwdDnwdPosMax_Val1 : Constant  Value=KeSMSwAcsMd7ThdRwRtStCshnFldUpwdDnwdPosMax_Val
  PA_KeSMSwAcsMd7ThdRwRtStCshnFldUpwdDnwdPosMin_Val1 : Constant  Value=KeSMSwAcsMd7ThdRwRtStCshnFldUpwdDnwdPosMin_Val
  PA_KeSMSwAcsMd7ThdRwRtStCshnFldUpwdDnwdPos_Val1 : Constant  Value=KeSMSwAcsMd7ThdRwRtStCshnFldUpwdDnwdPos_Val
  Subsystem : Subsystem
  Terminator_1 : Terminator
  Terminator_3 : Terminator
  Terminator_4 : Terminator
  EZER3RCshnFldTrgtPosCalib_TrgtPosArray_write : Outport  VectorParamsAs1DForOutWhenUnconnected=off
      settings: EnsureOutportIsVirtual=on
  LugRR3RCshnFldTrgtPosCalib_TrgtPosArray_write : Outport  Port=2  VectorParamsAs1DForOutWhenUnconnected=off
      settings: EnsureOutportIsVirtual=on
  Md53CshnFldTrgtPosCalib_TrgtPosArray_write : Outport  Port=3  VectorParamsAs1DForOutWhenUnconnected=off
      settings: EnsureOutportIsVirtual=on
  Md56R3RCshnFldTrgtPosCalib_TrgtPosArray_write : Outport  Port=4  VectorParamsAs1DForOutWhenUnconnected=off
      settings: EnsureOutportIsVirtual=on
  Md28R3RCshnFldTrgtPosCalib_TrgtPosArray_write : Outport  Port=5  VectorParamsAs1DForOutWhenUnconnected=off
  wires:
  StNumFlg_Is6s7s_read/1 -> Terminator_3/1
  StNumFlg_Is4s_read/1 -> Terminator_1/1
  StNumFlg_Is7s_read/1 -> Terminator_4/1
  Subsystem/1(EZER3RCshnFldTrgtPosCalib_TrgtPosArray_write) -> EZER3RCshnFldTrgtPosCalib_TrgtPosArray_write/1
  StNumFlg_Is6s_read/1 -> Subsystem/1(StNumFlg_Is6s_read)
  Subsystem/2(LugRR3RCshnFldTrgtPosCalib_TrgtPosArray_write) -> LugRR3RCshnFldTrgtPosCalib_TrgtPosArray_write/1
  Subsystem/3(Md53CshnFldTrgtPosCalib_TrgtPosArray_write) -> Md53CshnFldTrgtPosCalib_TrgtPosArray_write/1
  Subsystem/4(Md56R3RCshnFldTrgtPosCalib_TrgtPosArray_write) -> Md56R3RCshnFldTrgtPosCalib_TrgtPosArray_write/1
  PA_KeSMSwAcsMd7ThdRwRtStCshnFldUpwdDnwdPosMin_Val1/1 -> Mux1/3
  PA_KeSMSwAcsMd7ThdRwRtStCshnFldUpwdDnwdPos_Val1/1 -> Mux1/1
  PA_KeSMSwAcsMd7ThdRwRtStCshnFldUpwdDnwdPosMax_Val1/1 -> Mux1/2
  Mux1/1 -> Md28R3RCshnFldTrgtPosCalib_TrgtPosArray_write/1

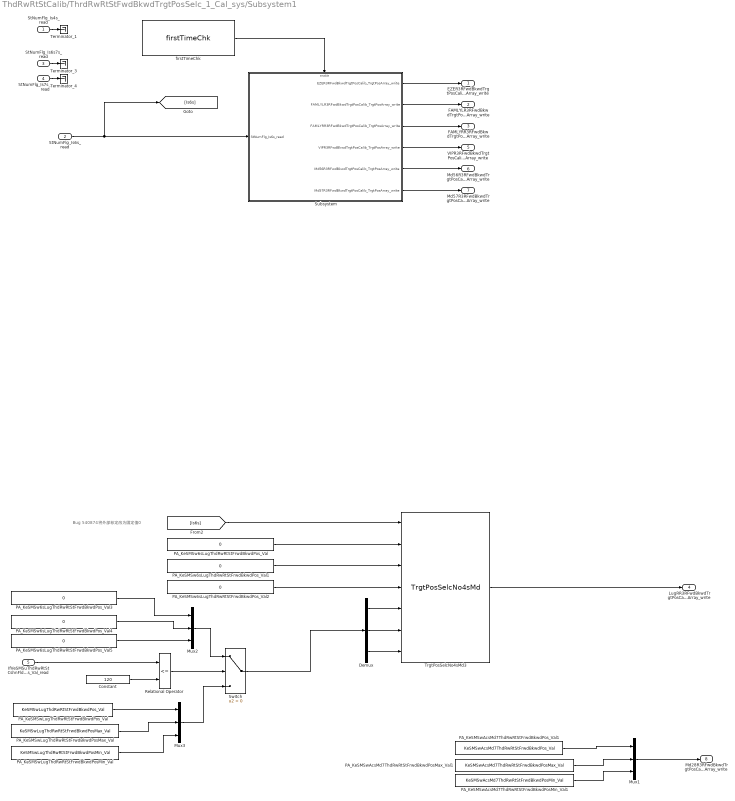
== system ThdRwRtStCalib/ThrdRwRtStFwdBkwdTrgtPosSelc_1_Cal_sys/Subsystem1 ==
  note: Bug 540874 将外部标定改为固定值0
  StNumFlg_Is4s_read : Inport
  StNumFlg_Is6s_read : Inport  Port=2
  StNumFlg_Is6s7s_read : Inport  Port=3
  StNumFlg_Is7s_read : Inport  Port=4
  IfVeSMSuThdRwRtStCshnFldUpwdDnwdPos_Val_read : Inport  Port=5
  Constant : Constant  Value=120  OutDataTypeStr=uint16
  Demux : Demux  Outputs=3
  Mux1 : Mux  Inputs=3
  Mux2 : Mux  Inputs=3
  Mux3 : Mux  Inputs=3
  PA_KeSMSw6sLugThdRwRtStFrwdBkwdPos_Val{,1..5} (6 alike) : Constant  Value=0  OutDataTypeStr=uint16
  PA_KeSMSwAcsMd7ThdRwRtStFrwdBkwdPosMax_Val1 : Constant  Value=KeSMSwAcsMd7ThdRwRtStFrwdBkwdPosMax_Val
  PA_KeSMSwAcsMd7ThdRwRtStFrwdBkwdPosMin_Val1 : Constant  Value=KeSMSwAcsMd7ThdRwRtStFrwdBkwdPosMin_Val
  PA_KeSMSwAcsMd7ThdRwRtStFrwdBkwdPos_Val1 : Constant  Value=KeSMSwAcsMd7ThdRwRtStFrwdBkwdPos_Val
  PA_KeSMSwLugThdRwRtStFrwdBkwdPosMax_Val : Constant  Value=KeSMSwLugThdRwRtStFrwdBkwdPosMax_Val
  PA_KeSMSwLugThdRwRtStFrwdBkwdPosMin_Val : Constant  Value=KeSMSwLugThdRwRtStFrwdBkwdPosMin_Val
  PA_KeSMSwLugThdRwRtStFrwdBkwdPos_Val : Constant  Value=KeSMSwLugThdRwRtStFrwdBkwdPos_Val
  Relational Operator : RelationalOperator  Operator=<=  OutDataTypeStr=boolean  RndMeth=Simplest  InputSameDT=off
  Subsystem : Subsystem
  Switch : Switch  Criteria=u2 > Threshold  SaturateOnIntegerOverflow=off  InputSameDT=off
  Terminator_1 : Terminator
  Terminator_3 : Terminator
  Terminator_4 : Terminator
  TrgtPosSelcNo4sMd3 : TrgtPosSelcLib/TrgtPosSelcNo4sMd  SystemSampleTime=-1  VariantActivationTime=update diagram  AllowFlexibleInterface=on  Latency=0  AutoFrameSizeCalculation=off
  firstTimeChk : TrgtPosSelcLib/firstTimeChk  SystemSampleTime=-1  VariantActivationTime=update diagram  AllowFlexibleInterface=on  Latency=0  AutoFrameSizeCalculation=off
  EZER3RFwdBkwdTrgtPosCalib_TrgtPosArray_write : Outport  VectorParamsAs1DForOutWhenUnconnected=off
      settings: EnsureOutportIsVirtual=on
  FAMLYLR3RFwdBkwdTrgtPosCalib_TrgtPosArray_write : Outport  Port=2  VectorParamsAs1DForOutWhenUnconnected=off
      settings: EnsureOutportIsVirtual=on
  FAMLYRR3RFwdBkwdTrgtPosCalib_TrgtPosArray_write : Outport  Port=3  VectorParamsAs1DForOutWhenUnconnected=off
      settings: EnsureOutportIsVirtual=on
  LugRR3RFwdBkwdTrgtPosCalib_TrgtPosArray_write : Outport  Port=4  VectorParamsAs1DForOutWhenUnconnected=off
      settings: EnsureOutportIsVirtual=on
  VIPR3RFwdBkwdTrgtPosCalib_TrgtPosArray_write : Outport  Port=5  VectorParamsAs1DForOutWhenUnconnected=off
      settings: EnsureOutportIsVirtual=on
  Md56R3RFwdBkwdTrgtPosCalib_TrgtPosArray_write : Outport  Port=6  VectorParamsAs1DForOutWhenUnconnected=off
      settings: EnsureOutportIsVirtual=on
  Md57R3RFwdBkwdTrgtPosCalib_TrgtPosArray_write : Outport  Port=7  VectorParamsAs1DForOutWhenUnconnected=off
      settings: EnsureOutportIsVirtual=on
  Md28R3RFwdBkwdTrgtPosCalib_TrgtPosArray_write : Outport  Port=8  VectorParamsAs1DForOutWhenUnconnected=off
  wires:
  StNumFlg_Is6s7s_read/1 -> Terminator_3/1
  StNumFlg_Is7s_read/1 -> Terminator_4/1
  Subsystem/4(VIPR3RFwdBkwdTrgtPosCalib_TrgtPosArray_write) -> VIPR3RFwdBkwdTrgtPosCalib_TrgtPosArray_write/1
  Subsystem/2(FAMLYLR3RFwdBkwdTrgtPosCalib_TrgtPosArray_write) -> FAMLYLR3RFwdBkwdTrgtPosCalib_TrgtPosArray_write/1
  StNumFlg_Is4s_read/1 -> Terminator_1/1
  Subsystem/3(FAMLYRR3RFwdBkwdTrgtPosCalib_TrgtPosArray_write) -> FAMLYRR3RFwdBkwdTrgtPosCalib_TrgtPosArray_write/1
  firstTimeChk/1 -> Subsystem/Enable
  StNumFlg_Is6s_read/1 -> [Is6s], Subsystem/1(StNumFlg_Is6s_read)
  TrgtPosSelcNo4sMd3/1 -> LugRR3RFwdBkwdTrgtPosCalib_TrgtPosArray_write/1
  Subsystem/1(EZER3RFwdBkwdTrgtPosCalib_TrgtPosArray_write) -> EZER3RFwdBkwdTrgtPosCalib_TrgtPosArray_write/1
  [Is6s] -> TrgtPosSelcNo4sMd3/1
  PA_KeSMSw6sLugThdRwRtStFrwdBkwdPos_Val1/1 -> TrgtPosSelcNo4sMd3/3
  PA_KeSMSw6sLugThdRwRtStFrwdBkwdPos_Val2/1 -> TrgtPosSelcNo4sMd3/4
  PA_KeSMSw6sLugThdRwRtStFrwdBkwdPos_Val/1 -> TrgtPosSelcNo4sMd3/2
  PA_KeSMSwLugThdRwRtStFrwdBkwdPos_Val/1 -> Mux3/1
  Demux/1 -> TrgtPosSelcNo4sMd3/5
  PA_KeSMSw6sLugThdRwRtStFrwdBkwdPos_Val4/1 -> Mux2/2
  Switch/1 -> Demux/1
  Mux3/1 -> Switch/3
  PA_KeSMSwLugThdRwRtStFrwdBkwdPosMin_Val/1 -> Mux3/3
  Mux2/1 -> Switch/1
  Relational Operator/1 -> Switch/2
  PA_KeSMSw6sLugThdRwRtStFrwdBkwdPos_Val5/1 -> Mux2/3
  Demux/3 -> TrgtPosSelcNo4sMd3/7
  PA_KeSMSwLugThdRwRtStFrwdBkwdPosMax_Val/1 -> Mux3/2
  PA_KeSMSw6sLugThdRwRtStFrwdBkwdPos_Val3/1 -> Mux2/1
  Demux/2 -> TrgtPosSelcNo4sMd3/6
  IfVeSMSuThdRwRtStCshnFldUpwdDnwdPos_Val_read/1 -> Relational Operator/1
  Constant/1 -> Relational Operator/2
  Subsystem/5(Md56R3RFwdBkwdTrgtPosCalib_TrgtPosArray_write) -> Md56R3RFwdBkwdTrgtPosCalib_TrgtPosArray_write/1
  Subsystem/6(Md57R3RFwdBkwdTrgtPosCalib_TrgtPosArray_write) -> Md57R3RFwdBkwdTrgtPosCalib_TrgtPosArray_write/1
  PA_KeSMSwAcsMd7ThdRwRtStFrwdBkwdPos_Val1/1 -> Mux1/1
  PA_KeSMSwAcsMd7ThdRwRtStFrwdBkwdPosMin_Val1/1 -> Mux1/3
  PA_KeSMSwAcsMd7ThdRwRtStFrwdBkwdPosMax_Val1/1 -> Mux1/2
  Mux1/1 -> Md28R3RFwdBkwdTrgtPosCalib_TrgtPosArray_write/1

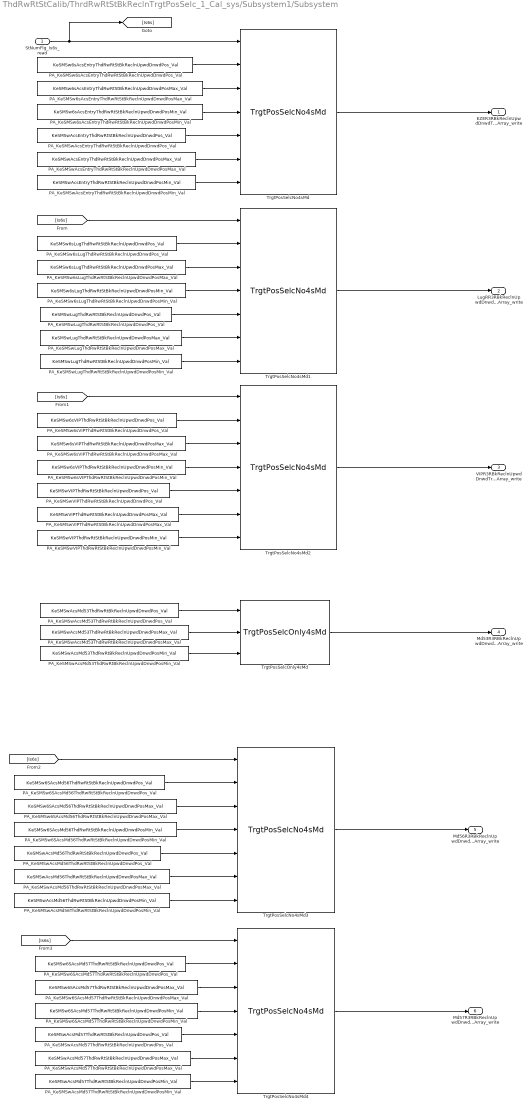
== system ThdRwRtStCalib/ThrdRwRtStBkReclnTrgtPosSelc_1_Cal_sys/Subsystem1/Subsystem ==
  StNumFlg_Is6s_read : Inport
  PA_KeSMSw6SAcsMd56ThdRwRtStBkReclnUpwdDnwdPosMax_Val : Constant  Value=KeSMSw6SAcsMd56ThdRwRtStBkReclnUpwdDnwdPosMax_Val
  PA_KeSMSw6SAcsMd56ThdRwRtStBkReclnUpwdDnwdPosMin_Val : Constant  Value=KeSMSw6SAcsMd56ThdRwRtStBkReclnUpwdDnwdPosMin_Val
  PA_KeSMSw6SAcsMd56ThdRwRtStBkReclnUpwdDnwdPos_Val : Constant  Value=KeSMSw6SAcsMd56ThdRwRtStBkReclnUpwdDnwdPos_Val
  PA_KeSMSw6SAcsMd57ThdRwRtStBkReclnUpwdDnwdPosMax_Val : Constant  Value=KeSMSw6SAcsMd57ThdRwRtStBkReclnUpwdDnwdPosMax_Val
  PA_KeSMSw6SAcsMd57ThdRwRtStBkReclnUpwdDnwdPosMin_Val : Constant  Value=KeSMSw6SAcsMd57ThdRwRtStBkReclnUpwdDnwdPosMin_Val
  PA_KeSMSw6SAcsMd57ThdRwRtStBkReclnUpwdDnwdPos_Val : Constant  Value=KeSMSw6SAcsMd57ThdRwRtStBkReclnUpwdDnwdPos_Val
  PA_KeSMSw6sAcsEntryThdRwRtStBkReclnUpwdDnwdPosMax_Val : Constant  Value=KeSMSw6sAcsEntryThdRwRtStBkReclnUpwdDnwdPosMax_Val
  PA_KeSMSw6sAcsEntryThdRwRtStBkReclnUpwdDnwdPosMin_Val : Constant  Value=KeSMSw6sAcsEntryThdRwRtStBkReclnUpwdDnwdPosMin_Val
  PA_KeSMSw6sAcsEntryThdRwRtStBkReclnUpwdDnwdPos_Val : Constant  Value=KeSMSw6sAcsEntryThdRwRtStBkReclnUpwdDnwdPos_Val
  PA_KeSMSw6sLugThdRwRtStBkReclnUpwdDnwdPosMax_Val : Constant  Value=KeSMSw6sLugThdRwRtStBkReclnUpwdDnwdPosMax_Val
  PA_KeSMSw6sLugThdRwRtStBkReclnUpwdDnwdPosMin_Val : Constant  Value=KeSMSw6sLugThdRwRtStBkReclnUpwdDnwdPosMin_Val
  PA_KeSMSw6sLugThdRwRtStBkReclnUpwdDnwdPos_Val : Constant  Value=KeSMSw6sLugThdRwRtStBkReclnUpwdDnwdPos_Val
  PA_KeSMSw6sVIPThdRwRtStBkReclnUpwdDnwdPosMax_Val : Constant  Value=KeSMSw6sVIPThdRwRtStBkReclnUpwdDnwdPosMax_Val
  PA_KeSMSw6sVIPThdRwRtStBkReclnUpwdDnwdPosMin_Val : Constant  Value=KeSMSw6sVIPThdRwRtStBkReclnUpwdDnwdPosMin_Val
  PA_KeSMSw6sVIPThdRwRtStBkReclnUpwdDnwdPos_Val : Constant  Value=KeSMSw6sVIPThdRwRtStBkReclnUpwdDnwdPos_Val
  PA_KeSMSwAcsEntryThdRwRtStBkReclnUpwdDnwdPosMax_Val : Constant  Value=KeSMSwAcsEntryThdRwRtStBkReclnUpwdDnwdPosMax_Val
  PA_KeSMSwAcsEntryThdRwRtStBkReclnUpwdDnwdPosMin_Val : Constant  Value=KeSMSwAcsEntryThdRwRtStBkReclnUpwdDnwdPosMin_Val
  PA_KeSMSwAcsEntryThdRwRtStBkReclnUpwdDnwdPos_Val : Constant  Value=KeSMSwAcsEntryThdRwRtStBkReclnUpwdDnwdPos_Val
  PA_KeSMSwAcsMd53ThdRwRtBkReclnUpwdDnwdPosMax_Val : Constant  Value=KeSMSwAcsMd53ThdRwRtBkReclnUpwdDnwdPosMax_Val
  PA_KeSMSwAcsMd53ThdRwRtBkReclnUpwdDnwdPosMin_Val : Constant  Value=KeSMSwAcsMd53ThdRwRtBkReclnUpwdDnwdPosMin_Val
  PA_KeSMSwAcsMd53ThdRwRtBkReclnUpwdDnwdPos_Val : Constant  Value=KeSMSwAcsMd53ThdRwRtBkReclnUpwdDnwdPos_Val
  PA_KeSMSwAcsMd56ThdRwRtStBkReclnUpwdDnwdPosMax_Val : Constant  Value=KeSMSwAcsMd56ThdRwRtStBkReclnUpwdDnwdPosMax_Val
  PA_KeSMSwAcsMd56ThdRwRtStBkReclnUpwdDnwdPosMin_Val : Constant  Value=KeSMSwAcsMd56ThdRwRtStBkReclnUpwdDnwdPosMin_Val
  PA_KeSMSwAcsMd56ThdRwRtStBkReclnUpwdDnwdPos_Val : Constant  Value=KeSMSwAcsMd56ThdRwRtStBkReclnUpwdDnwdPos_Val
  PA_KeSMSwAcsMd57ThdRwRtStBkReclnUpwdDnwdPosMax_Val : Constant  Value=KeSMSwAcsMd57ThdRwRtStBkReclnUpwdDnwdPosMax_Val
  PA_KeSMSwAcsMd57ThdRwRtStBkReclnUpwdDnwdPosMin_Val : Constant  Value=KeSMSwAcsMd57ThdRwRtStBkReclnUpwdDnwdPosMin_Val
  PA_KeSMSwAcsMd57ThdRwRtStBkReclnUpwdDnwdPos_Val : Constant  Value=KeSMSwAcsMd57ThdRwRtStBkReclnUpwdDnwdPos_Val
  PA_KeSMSwLugThdRwRtStBkReclnUpwdDnwdPosMax_Val : Constant  Value=KeSMSwLugThdRwRtStBkReclnUpwdDnwdPosMax_Val
  PA_KeSMSwLugThdRwRtStBkReclnUpwdDnwdPosMin_Val : Constant  Value=KeSMSwLugThdRwRtStBkReclnUpwdDnwdPosMin_Val
  PA_KeSMSwLugThdRwRtStBkReclnUpwdDnwdPos_Val : Constant  Value=KeSMSwLugThdRwRtStBkReclnUpwdDnwdPos_Val
  PA_KeSMSwVIPThdRwRtStBkReclnUpwdDnwdPosMax_Val : Constant  Value=KeSMSwVIPThdRwRtStBkReclnUpwdDnwdPosMax_Val
  PA_KeSMSwVIPThdRwRtStBkReclnUpwdDnwdPosMin_Val : Constant  Value=KeSMSwVIPThdRwRtStBkReclnUpwdDnwdPosMin_Val
  PA_KeSMSwVIPThdRwRtStBkReclnUpwdDnwdPos_Val : Constant  Value=KeSMSwVIPThdRwRtStBkReclnUpwdDnwdPos_Val
  TrgtPosSelcNo4sMd{,1..4} (5 alike) : TrgtPosSelcLib/TrgtPosSelcNo4sMd  SystemSampleTime=-1  VariantActivationTime=update diagram  AllowFlexibleInterface=on  Latency=0  AutoFrameSizeCalculation=off
  TrgtPosSelcOnly4sMd : TrgtPosSelcLib/TrgtPosSelcOnly4sMd  SystemSampleTime=-1  VariantActivationTime=update diagram  AllowFlexibleInterface=on  Latency=0  AutoFrameSizeCalculation=off
  EZER3RBkReclnUpwdDnwdTrgtPosCalib_TrgtPosArray_write : Outport  VectorParamsAs1DForOutWhenUnconnected=off
      settings: EnsureOutportIsVirtual=on
  LugRR3RBkReclnUpwdDnwdTrgtPosCalib_TrgtPosArray_write : Outport  Port=2  VectorParamsAs1DForOutWhenUnconnected=off
      settings: EnsureOutportIsVirtual=on
  VIPR3RBkReclnUpwdDnwdTrgtPosCalib_TrgtPosArray_write : Outport  Port=3  VectorParamsAs1DForOutWhenUnconnected=off
      settings: EnsureOutportIsVirtual=on
  Md53R3RBkReclnUpwdDnwdTrgtPosCalib_TrgtPosArray_write : Outport  Port=4  VectorParamsAs1DForOutWhenUnconnected=off
      settings: EnsureOutportIsVirtual=on
  Md56R3RBkReclnUpwdDnwdTrgtPosCalib_TrgtPosArray_write : Outport  Port=5  VectorParamsAs1DForOutWhenUnconnected=off
      settings: EnsureOutportIsVirtual=on
  Md57R3RBkReclnUpwdDnwdTrgtPosCalib_TrgtPosArray_write : Outport  Port=6  VectorParamsAs1DForOutWhenUnconnected=off
      settings: EnsureOutportIsVirtual=on
  wires:
  TrgtPosSelcNo4sMd1/1 -> LugRR3RBkReclnUpwdDnwdTrgtPosCalib_TrgtPosArray_write/1
  StNumFlg_Is6s_read/1 -> [Is6s], TrgtPosSelcNo4sMd/1
  TrgtPosSelcNo4sMd/1 -> EZER3RBkReclnUpwdDnwdTrgtPosCalib_TrgtPosArray_write/1
  TrgtPosSelcNo4sMd2/1 -> VIPR3RBkReclnUpwdDnwdTrgtPosCalib_TrgtPosArray_write/1
  PA_KeSMSw6sAcsEntryThdRwRtStBkReclnUpwdDnwdPosMax_Val/1 -> TrgtPosSelcNo4sMd/3
  PA_KeSMSw6sAcsEntryThdRwRtStBkReclnUpwdDnwdPos_Val/1 -> TrgtPosSelcNo4sMd/2
  PA_KeSMSw6sAcsEntryThdRwRtStBkReclnUpwdDnwdPosMin_Val/1 -> TrgtPosSelcNo4sMd/4
  [Is6s] -> TrgtPosSelcNo4sMd1/1
  [Is6s] -> TrgtPosSelcNo4sMd2/1
  PA_KeSMSw6sLugThdRwRtStBkReclnUpwdDnwdPosMax_Val/1 -> TrgtPosSelcNo4sMd1/3
  PA_KeSMSw6sLugThdRwRtStBkReclnUpwdDnwdPos_Val/1 -> TrgtPosSelcNo4sMd1/2
  PA_KeSMSw6sLugThdRwRtStBkReclnUpwdDnwdPosMin_Val/1 -> TrgtPosSelcNo4sMd1/4
  PA_KeSMSw6sVIPThdRwRtStBkReclnUpwdDnwdPosMax_Val/1 -> TrgtPosSelcNo4sMd2/3
  PA_KeSMSw6sVIPThdRwRtStBkReclnUpwdDnwdPos_Val/1 -> TrgtPosSelcNo4sMd2/2
  PA_KeSMSw6sVIPThdRwRtStBkReclnUpwdDnwdPosMin_Val/1 -> TrgtPosSelcNo4sMd2/4
  PA_KeSMSwAcsEntryThdRwRtStBkReclnUpwdDnwdPosMax_Val/1 -> TrgtPosSelcNo4sMd/6
  PA_KeSMSwAcsEntryThdRwRtStBkReclnUpwdDnwdPos_Val/1 -> TrgtPosSelcNo4sMd/5
  PA_KeSMSwAcsEntryThdRwRtStBkReclnUpwdDnwdPosMin_Val/1 -> TrgtPosSelcNo4sMd/7
  PA_KeSMSwLugThdRwRtStBkReclnUpwdDnwdPosMax_Val/1 -> TrgtPosSelcNo4sMd1/6
  PA_KeSMSwLugThdRwRtStBkReclnUpwdDnwdPosMin_Val/1 -> TrgtPosSelcNo4sMd1/7
  PA_KeSMSwLugThdRwRtStBkReclnUpwdDnwdPos_Val/1 -> TrgtPosSelcNo4sMd1/5
  PA_KeSMSwVIPThdRwRtStBkReclnUpwdDnwdPosMax_Val/1 -> TrgtPosSelcNo4sMd2/6
  PA_KeSMSwVIPThdRwRtStBkReclnUpwdDnwdPos_Val/1 -> TrgtPosSelcNo4sMd2/5
  PA_KeSMSwVIPThdRwRtStBkReclnUpwdDnwdPosMin_Val/1 -> TrgtPosSelcNo4sMd2/7
  PA_KeSMSwAcsMd53ThdRwRtBkReclnUpwdDnwdPosMin_Val/1 -> TrgtPosSelcOnly4sMd/3
  PA_KeSMSwAcsMd53ThdRwRtBkReclnUpwdDnwdPosMax_Val/1 -> TrgtPosSelcOnly4sMd/2
  PA_KeSMSwAcsMd53ThdRwRtBkReclnUpwdDnwdPos_Val/1 -> TrgtPosSelcOnly4sMd/1
  TrgtPosSelcOnly4sMd/1 -> Md53R3RBkReclnUpwdDnwdTrgtPosCalib_TrgtPosArray_write/1
  TrgtPosSelcNo4sMd3/1 -> Md56R3RBkReclnUpwdDnwdTrgtPosCalib_TrgtPosArray_write/1
  PA_KeSMSwAcsMd56ThdRwRtStBkReclnUpwdDnwdPosMin_Val/1 -> TrgtPosSelcNo4sMd3/7
  PA_KeSMSwAcsMd56ThdRwRtStBkReclnUpwdDnwdPosMax_Val/1 -> TrgtPosSelcNo4sMd3/6
  PA_KeSMSwAcsMd56ThdRwRtStBkReclnUpwdDnwdPos_Val/1 -> TrgtPosSelcNo4sMd3/5
  PA_KeSMSw6SAcsMd56ThdRwRtStBkReclnUpwdDnwdPosMin_Val/1 -> TrgtPosSelcNo4sMd3/4
  PA_KeSMSw6SAcsMd56ThdRwRtStBkReclnUpwdDnwdPosMax_Val/1 -> TrgtPosSelcNo4sMd3/3
  PA_KeSMSw6SAcsMd56ThdRwRtStBkReclnUpwdDnwdPos_Val/1 -> TrgtPosSelcNo4sMd3/2
  [Is6s] -> TrgtPosSelcNo4sMd3/1
  [Is6s] -> TrgtPosSelcNo4sMd4/1
  TrgtPosSelcNo4sMd4/1 -> Md57R3RBkReclnUpwdDnwdTrgtPosCalib_TrgtPosArray_write/1
  PA_KeSMSw6SAcsMd57ThdRwRtStBkReclnUpwdDnwdPosMax_Val/1 -> TrgtPosSelcNo4sMd4/3
  PA_KeSMSw6SAcsMd57ThdRwRtStBkReclnUpwdDnwdPos_Val/1 -> TrgtPosSelcNo4sMd4/2
  PA_KeSMSw6SAcsMd57ThdRwRtStBkReclnUpwdDnwdPosMin_Val/1 -> TrgtPosSelcNo4sMd4/4
  PA_KeSMSwAcsMd57ThdRwRtStBkReclnUpwdDnwdPosMax_Val/1 -> TrgtPosSelcNo4sMd4/6
  PA_KeSMSwAcsMd57ThdRwRtStBkReclnUpwdDnwdPos_Val/1 -> TrgtPosSelcNo4sMd4/5
  PA_KeSMSwAcsMd57ThdRwRtStBkReclnUpwdDnwdPosMin_Val/1 -> TrgtPosSelcNo4sMd4/7

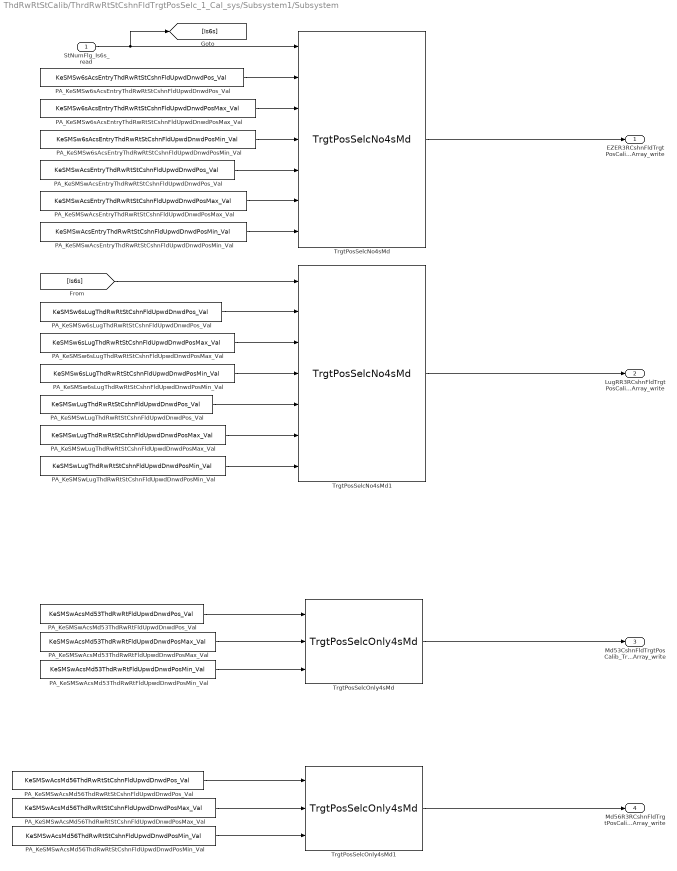
== system ThdRwRtStCalib/ThrdRwRtStCshnFldTrgtPosSelc_1_Cal_sys/Subsystem1/Subsystem ==
  StNumFlg_Is6s_read : Inport
  PA_KeSMSw6sAcsEntryThdRwRtStCshnFldUpwdDnwdPosMax_Val : Constant  Value=KeSMSw6sAcsEntryThdRwRtStCshnFldUpwdDnwdPosMax_Val
  PA_KeSMSw6sAcsEntryThdRwRtStCshnFldUpwdDnwdPosMin_Val : Constant  Value=KeSMSw6sAcsEntryThdRwRtStCshnFldUpwdDnwdPosMin_Val
  PA_KeSMSw6sAcsEntryThdRwRtStCshnFldUpwdDnwdPos_Val : Constant  Value=KeSMSw6sAcsEntryThdRwRtStCshnFldUpwdDnwdPos_Val
  PA_KeSMSw6sLugThdRwRtStCshnFldUpwdDnwdPosMax_Val : Constant  Value=KeSMSw6sLugThdRwRtStCshnFldUpwdDnwdPosMax_Val
  PA_KeSMSw6sLugThdRwRtStCshnFldUpwdDnwdPosMin_Val : Constant  Value=KeSMSw6sLugThdRwRtStCshnFldUpwdDnwdPosMin_Val
  PA_KeSMSw6sLugThdRwRtStCshnFldUpwdDnwdPos_Val : Constant  Value=KeSMSw6sLugThdRwRtStCshnFldUpwdDnwdPos_Val
  PA_KeSMSwAcsEntryThdRwRtStCshnFldUpwdDnwdPosMax_Val : Constant  Value=KeSMSwAcsEntryThdRwRtStCshnFldUpwdDnwdPosMax_Val
  PA_KeSMSwAcsEntryThdRwRtStCshnFldUpwdDnwdPosMin_Val : Constant  Value=KeSMSwAcsEntryThdRwRtStCshnFldUpwdDnwdPosMin_Val
  PA_KeSMSwAcsEntryThdRwRtStCshnFldUpwdDnwdPos_Val : Constant  Value=KeSMSwAcsEntryThdRwRtStCshnFldUpwdDnwdPos_Val
  PA_KeSMSwAcsMd53ThdRwRtFldUpwdDnwdPosMax_Val : Constant  Value=KeSMSwAcsMd53ThdRwRtFldUpwdDnwdPosMax_Val
  PA_KeSMSwAcsMd53ThdRwRtFldUpwdDnwdPosMin_Val : Constant  Value=KeSMSwAcsMd53ThdRwRtFldUpwdDnwdPosMin_Val
  PA_KeSMSwAcsMd53ThdRwRtFldUpwdDnwdPos_Val : Constant  Value=KeSMSwAcsMd53ThdRwRtFldUpwdDnwdPos_Val
  PA_KeSMSwAcsMd56ThdRwRtStCshnFldUpwdDnwdPosMax_Val : Constant  Value=KeSMSwAcsMd56ThdRwRtStCshnFldUpwdDnwdPosMax_Val
  PA_KeSMSwAcsMd56ThdRwRtStCshnFldUpwdDnwdPosMin_Val : Constant  Value=KeSMSwAcsMd56ThdRwRtStCshnFldUpwdDnwdPosMin_Val
  PA_KeSMSwAcsMd56ThdRwRtStCshnFldUpwdDnwdPos_Val : Constant  Value=KeSMSwAcsMd56ThdRwRtStCshnFldUpwdDnwdPos_Val
  PA_KeSMSwLugThdRwRtStCshnFldUpwdDnwdPosMax_Val : Constant  Value=KeSMSwLugThdRwRtStCshnFldUpwdDnwdPosMax_Val
  PA_KeSMSwLugThdRwRtStCshnFldUpwdDnwdPosMin_Val : Constant  Value=KeSMSwLugThdRwRtStCshnFldUpwdDnwdPosMin_Val
  PA_KeSMSwLugThdRwRtStCshnFldUpwdDnwdPos_Val : Constant  Value=KeSMSwLugThdRwRtStCshnFldUpwdDnwdPos_Val
  TrgtPosSelcNo4sMd : TrgtPosSelcLib/TrgtPosSelcNo4sMd  SystemSampleTime=-1  VariantActivationTime=update diagram  AllowFlexibleInterface=on  Latency=0  AutoFrameSizeCalculation=off
  TrgtPosSelcNo4sMd1 : TrgtPosSelcLib/TrgtPosSelcNo4sMd  SystemSampleTime=-1  VariantActivationTime=update diagram  AllowFlexibleInterface=on  Latency=0  AutoFrameSizeCalculation=off
  TrgtPosSelcOnly4sMd : TrgtPosSelcLib/TrgtPosSelcOnly4sMd  SystemSampleTime=-1  VariantActivationTime=update diagram  AllowFlexibleInterface=on  Latency=0  AutoFrameSizeCalculation=off
  TrgtPosSelcOnly4sMd1 : TrgtPosSelcLib/TrgtPosSelcOnly4sMd  SystemSampleTime=-1  VariantActivationTime=update diagram  AllowFlexibleInterface=on  Latency=0  AutoFrameSizeCalculation=off
  EZER3RCshnFldTrgtPosCalib_TrgtPosArray_write : Outport  VectorParamsAs1DForOutWhenUnconnected=off
      settings: EnsureOutportIsVirtual=on
  LugRR3RCshnFldTrgtPosCalib_TrgtPosArray_write : Outport  Port=2  VectorParamsAs1DForOutWhenUnconnected=off
      settings: EnsureOutportIsVirtual=on
  Md53CshnFldTrgtPosCalib_TrgtPosArray_write : Outport  Port=3  VectorParamsAs1DForOutWhenUnconnected=off
      settings: EnsureOutportIsVirtual=on
  Md56R3RCshnFldTrgtPosCalib_TrgtPosArray_write : Outport  Port=4  VectorParamsAs1DForOutWhenUnconnected=off
      settings: EnsureOutportIsVirtual=on
  wires:
  StNumFlg_Is6s_read/1 -> [Is6s], TrgtPosSelcNo4sMd/1
  TrgtPosSelcNo4sMd/1 -> EZER3RCshnFldTrgtPosCalib_TrgtPosArray_write/1
  TrgtPosSelcNo4sMd1/1 -> LugRR3RCshnFldTrgtPosCalib_TrgtPosArray_write/1
  PA_KeSMSw6sAcsEntryThdRwRtStCshnFldUpwdDnwdPosMax_Val/1 -> TrgtPosSelcNo4sMd/3
  PA_KeSMSw6sAcsEntryThdRwRtStCshnFldUpwdDnwdPos_Val/1 -> TrgtPosSelcNo4sMd/2
  PA_KeSMSw6sAcsEntryThdRwRtStCshnFldUpwdDnwdPosMin_Val/1 -> TrgtPosSelcNo4sMd/4
  PA_KeSMSwAcsEntryThdRwRtStCshnFldUpwdDnwdPosMax_Val/1 -> TrgtPosSelcNo4sMd/6
  PA_KeSMSwAcsEntryThdRwRtStCshnFldUpwdDnwdPosMin_Val/1 -> TrgtPosSelcNo4sMd/7
  PA_KeSMSwAcsEntryThdRwRtStCshnFldUpwdDnwdPos_Val/1 -> TrgtPosSelcNo4sMd/5
  [Is6s] -> TrgtPosSelcNo4sMd1/1
  PA_KeSMSw6sLugThdRwRtStCshnFldUpwdDnwdPosMax_Val/1 -> TrgtPosSelcNo4sMd1/3
  PA_KeSMSw6sLugThdRwRtStCshnFldUpwdDnwdPos_Val/1 -> TrgtPosSelcNo4sMd1/2
  PA_KeSMSw6sLugThdRwRtStCshnFldUpwdDnwdPosMin_Val/1 -> TrgtPosSelcNo4sMd1/4
  PA_KeSMSwLugThdRwRtStCshnFldUpwdDnwdPosMin_Val/1 -> TrgtPosSelcNo4sMd1/7
  PA_KeSMSwLugThdRwRtStCshnFldUpwdDnwdPosMax_Val/1 -> TrgtPosSelcNo4sMd1/6
  PA_KeSMSwLugThdRwRtStCshnFldUpwdDnwdPos_Val/1 -> TrgtPosSelcNo4sMd1/5
  PA_KeSMSwAcsMd53ThdRwRtFldUpwdDnwdPos_Val/1 -> TrgtPosSelcOnly4sMd/1
  PA_KeSMSwAcsMd53ThdRwRtFldUpwdDnwdPosMax_Val/1 -> TrgtPosSelcOnly4sMd/2
  PA_KeSMSwAcsMd53ThdRwRtFldUpwdDnwdPosMin_Val/1 -> TrgtPosSelcOnly4sMd/3
  TrgtPosSelcOnly4sMd/1 -> Md53CshnFldTrgtPosCalib_TrgtPosArray_write/1
  TrgtPosSelcOnly4sMd1/1 -> Md56R3RCshnFldTrgtPosCalib_TrgtPosArray_write/1
  PA_KeSMSwAcsMd56ThdRwRtStCshnFldUpwdDnwdPosMin_Val/1 -> TrgtPosSelcOnly4sMd1/3
  PA_KeSMSwAcsMd56ThdRwRtStCshnFldUpwdDnwdPosMax_Val/1 -> TrgtPosSelcOnly4sMd1/2
  PA_KeSMSwAcsMd56ThdRwRtStCshnFldUpwdDnwdPos_Val/1 -> TrgtPosSelcOnly4sMd1/1
